simulink model "Selfmade_model_robot"  (R2024b)
settings: Solver=VariableStepAuto  StartTime=0.0  StopTime=10.0  RelTol=1e-3
values from neighbouring files (symbols this model uses):
  ua2tau = (2*gbox.N*mot.Kt/mot.R)*[1;-1]    [lab4_model_startup.m]
undefined symbols (not defined in the file or in its folder): drv, g, gbox, model, ms22g, sens, Ts, wheel
settings Model: Creator=bmm1  LastModifiedBy=pries

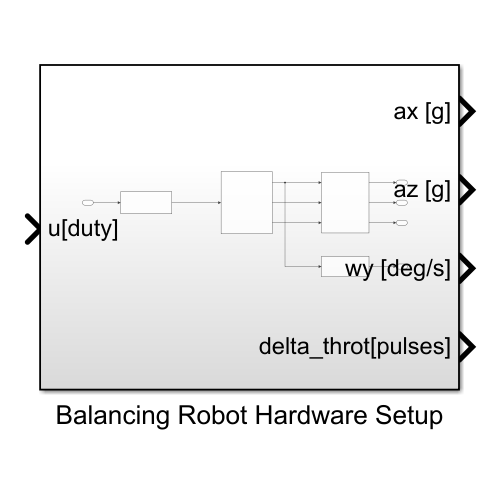
[thumbnail: Simulink's stored preview of the top-level diagram]
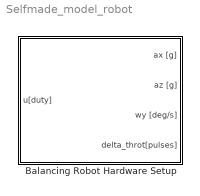
== system Selfmade_model_robot ==
  Balancing Robot Hardware Setup : Subsystem

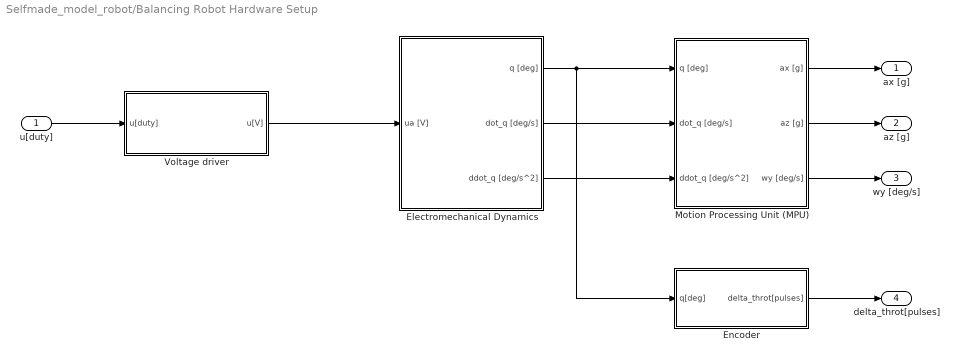
== system Selfmade_model_robot/Balancing Robot Hardware Setup ==
  u[duty] : Inport
  Electromechanical Dynamics : Subsystem
  Encoder : Subsystem
  Motion Processing Unit (MPU) : Subsystem
  Voltage driver : Subsystem
  ax [g] : Outport
  az [g] : Outport  Port=2
  wy [deg/s] : Outport  Port=3
  delta_throt[pulses] : Outport  Port=4
  wires:
  Voltage driver/1(u[V]) -> Electromechanical Dynamics/1(ua [V])
  Electromechanical Dynamics/1(q [deg]) -> Encoder/1(q[deg]), Motion Processing Unit (MPU)/1(q [deg])
  u[duty]/1 -> Voltage driver/1(u[duty])
  Electromechanical Dynamics/3(ddot_q [deg/s^2]) -> Motion Processing Unit (MPU)/3(ddot_q [deg/s^2])
  Motion Processing Unit (MPU)/3(wy [deg/s]) -> wy [deg/s]/1
  Electromechanical Dynamics/2(dot_q [deg/s]) -> Motion Processing Unit (MPU)/2(dot_q [deg/s])
  Motion Processing Unit (MPU)/2(az [g]) -> az [g]/1
  Motion Processing Unit (MPU)/1(ax [g]) -> ax [g]/1
  Encoder/1(delta_throt[pulses]) -> delta_throt[pulses]/1

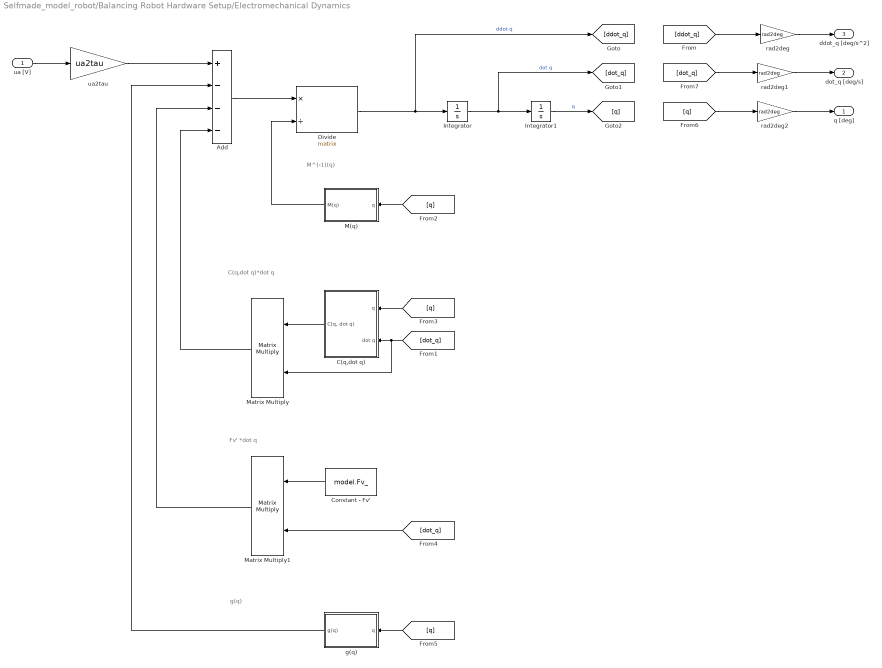
== system Selfmade_model_robot/Balancing Robot Hardware Setup/Electromechanical Dynamics ==
  note: g(q)
  note: Fv' *dot q
  note: C(q,dot q)*dot q
  note: M^(-1)(q)
  ua [V] : Inport
  Add : Sum  Inputs=+---
  C(q,dot q) : Subsystem
  Constant - Fv' : Constant  Value=model.Fv_
  Divide : Product  Inputs=*/  Multiplication=Matrix(*)
  Integrator : Integrator
  Integrator1 : Integrator
  M(q) : Subsystem
  Matrix Multiply : Product  Multiplication=Matrix(*)
  Matrix Multiply1 : Product  Multiplication=Matrix(*)
  g(q) : Subsystem
  rad2deg : Gain  Gain=rad2deg
  rad2deg1 : Gain  Gain=rad2deg
  rad2deg2 : Gain  Gain=rad2deg
  ua2tau : Gain  Gain=ua2tau
  q [deg] : Outport
  dot_q [deg/s] : Outport  Port=2
  ddot_q [deg/s^2] : Outport  Port=3
  wires:
  ua [V]/1 -> ua2tau/1
  ua2tau/1 -> Add/1
  Add/1 -> Divide/1
  Divide/1 -> [ddot_q], Integrator/1  "ddot q"
  Integrator/1 -> [dot_q], Integrator1/1  "dot q"
  Integrator1/1 -> [q]  "q"
  [q] -> M(q)/1(q)
  M(q)/1(M(q)) -> Divide/2
  C(q,dot q)/1("C(q, dot q)") -> Matrix Multiply/1
  [dot_q] -> Matrix Multiply/2, C(q,dot q)/2(dot q)
  [q] -> C(q,dot q)/1(q)
  Constant - Fv'/1 -> Matrix Multiply1/1
  [dot_q] -> Matrix Multiply1/2
  [q] -> g(q)/1(q)
  Matrix Multiply/1 -> Add/4
  Matrix Multiply1/1 -> Add/3
  g(q)/1(g(q)) -> Add/2
  [ddot_q] -> rad2deg/1
  [dot_q] -> rad2deg1/1
  [q] -> rad2deg2/1
  rad2deg2/1 -> q [deg]/1
  rad2deg/1 -> ddot_q [deg/s^2]/1
  rad2deg1/1 -> dot_q [deg/s]/1

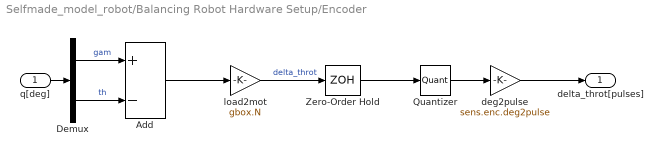
== system Selfmade_model_robot/Balancing Robot Hardware Setup/Encoder ==
  q[deg] : Inport
  Add : Sum  Inputs=+-
  Demux : Demux  Outputs=2
  Quantizer : Quantizer  QuantizationInterval=sens.enc.pulse2deg
  Zero-Order Hold : ZeroOrderHold  SampleTime=Ts
  deg2pulse : Gain  Gain=sens.enc.deg2pulse
  load2mot : Gain  Gain=gbox.N
  delta_throt[pulses] : Outport
  wires:
  Add/1 -> load2mot/1
  Zero-Order Hold/1 -> Quantizer/1
  q[deg]/1 -> Demux/1
  Demux/2 -> Add/2  "th"
  Quantizer/1 -> deg2pulse/1
  Demux/1 -> Add/1  "gam"
  deg2pulse/1 -> delta_throt[pulses]/1
  load2mot/1 -> Zero-Order Hold/1  "delta_throt"

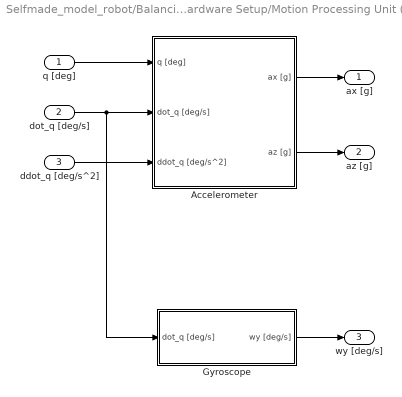
== system Selfmade_model_robot/Balancing Robot Hardware Setup/Motion Processing Unit (MPU) ==
  q [deg] : Inport
  dot_q [deg/s] : Inport  Port=2
  ddot_q [deg/s^2] : Inport  Port=3
  Accelerometer : Subsystem
  Gyroscope : Subsystem
  ax [g] : Outport
  az [g] : Outport  Port=2
  wy [deg/s] : Outport  Port=3
  wires:
  Gyroscope/1(wy [deg/s]) -> wy [deg/s]/1
  ddot_q [deg/s^2]/1 -> Accelerometer/3(ddot_q [deg/s^2])
  q [deg]/1 -> Accelerometer/1(q [deg])
  Accelerometer/1(ax [g]) -> ax [g]/1
  dot_q [deg/s]/1 -> Gyroscope/1(dot_q [deg/s]), Accelerometer/2(dot_q [deg/s])
  Accelerometer/2(az [g]) -> az [g]/1

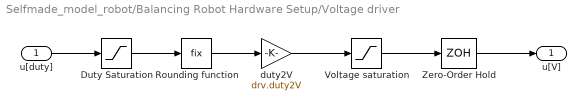
== system Selfmade_model_robot/Balancing Robot Hardware Setup/Voltage driver ==
  u[duty] : Inport
  Duty Saturation : Saturate  UpperLimit=drv.dutymax  LowerLimit=-drv.dutymax
  Rounding function : Rounding  Operator=fix
  Voltage saturation : Saturate  UpperLimit=drv.Vbus  LowerLimit=-drv.Vbus
  Zero-Order Hold : ZeroOrderHold  SampleTime=Ts
  duty2V : Gain  Gain=drv.duty2V
  u[V] : Outport
  wires:
  Voltage saturation/1 -> Zero-Order Hold/1
  duty2V/1 -> Voltage saturation/1
  Rounding function/1 -> duty2V/1
  Zero-Order Hold/1 -> u[V]/1
  Duty Saturation/1 -> Rounding function/1
  u[duty]/1 -> Duty Saturation/1

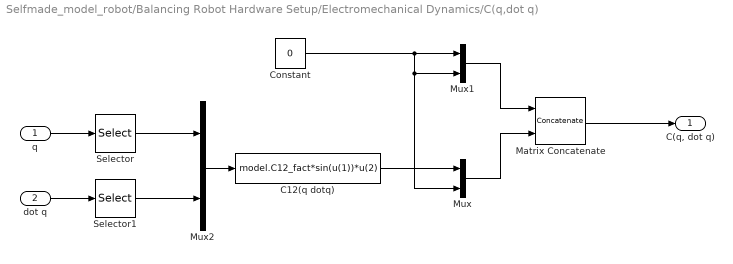
== system Selfmade_model_robot/Balancing Robot Hardware Setup/Electromechanical Dynamics/C(q,dot q) ==
  q : Inport
  dot q : Inport  Port=2
  C12(q dotq) : Fcn  Expr=model.C12_fact*sin(u(1))*u(2)
  Constant : Constant  Value=0
  Matrix Concatenate : Concatenate  Mode=Multidimensional array  ConcatenateDimension=2
  Mux : Mux  Inputs=2
  Mux1 : Mux  Inputs=2
  Mux2 : Mux  Inputs=2
  Selector : Selector  InputPortWidth=2  IndexOptions=Index vector (dialog)  Indices=2  OutputSizes=1
  Selector1 : Selector  InputPortWidth=2  IndexOptions=Index vector (dialog)  Indices=2  OutputSizes=1
  "C(q, dot q)" : Outport
  wires:
  Matrix Concatenate/1 -> "C(q, dot q)"/1
  Mux/1 -> Matrix Concatenate/2
  Mux1/1 -> Matrix Concatenate/1
  Selector/1 -> Mux2/1
  q/1 -> Selector/1
  dot q/1 -> Selector1/1
  Constant/1 -> Mux/2, Mux1/2, Mux1/1
  Selector1/1 -> Mux2/2
  Mux2/1 -> C12(q dotq)/1
  C12(q dotq)/1 -> Mux/1

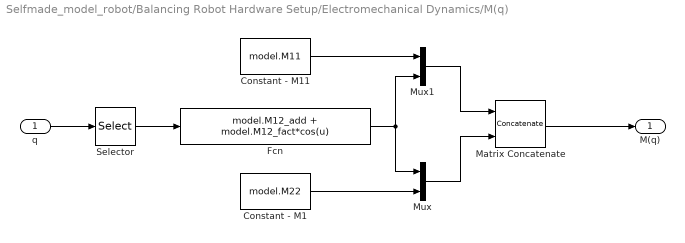
== system Selfmade_model_robot/Balancing Robot Hardware Setup/Electromechanical Dynamics/M(q) ==
  q : Inport
  Constant - M1 : Constant  Value=model.M22
  Constant - M11 : Constant  Value=model.M11
  Fcn : Fcn  Expr=model.M12_add + model.M12_fact*cos(u)
  Matrix Concatenate : Concatenate  Mode=Multidimensional array  ConcatenateDimension=2
  Mux : Mux  Inputs=2
  Mux1 : Mux  Inputs=2
  Selector : Selector  InputPortWidth=2  IndexOptions=Index vector (dialog)  Indices=2  OutputSizes=1
  M(q) : Outport
  wires:
  q/1 -> Selector/1
  Selector/1 -> Fcn/1
  Constant - M1/1 -> Mux/2
  Constant - M11/1 -> Mux1/1
  Fcn/1 -> Mux/1, Mux1/2
  Mux1/1 -> Matrix Concatenate/1
  Mux/1 -> Matrix Concatenate/2
  Matrix Concatenate/1 -> M(q)/1

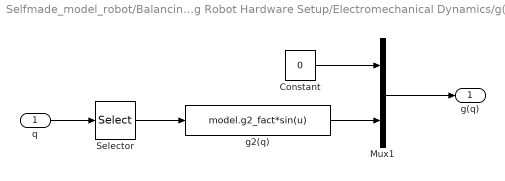
== system Selfmade_model_robot/Balancing Robot Hardware Setup/Electromechanical Dynamics/g(q) ==
  q : Inport
  Constant : Constant  Value=0
  Mux1 : Mux  Inputs=2
  Selector : Selector  InputPortWidth=2  IndexOptions=Index vector (dialog)  Indices=2  OutputSizes=1
  g2(q) : Fcn  Expr=model.g2_fact*sin(u)
  g(q) : Outport
  wires:
  Selector/1 -> g2(q)/1
  Constant/1 -> Mux1/1
  q/1 -> Selector/1
  g2(q)/1 -> Mux1/2
  Mux1/1 -> g(q)/1

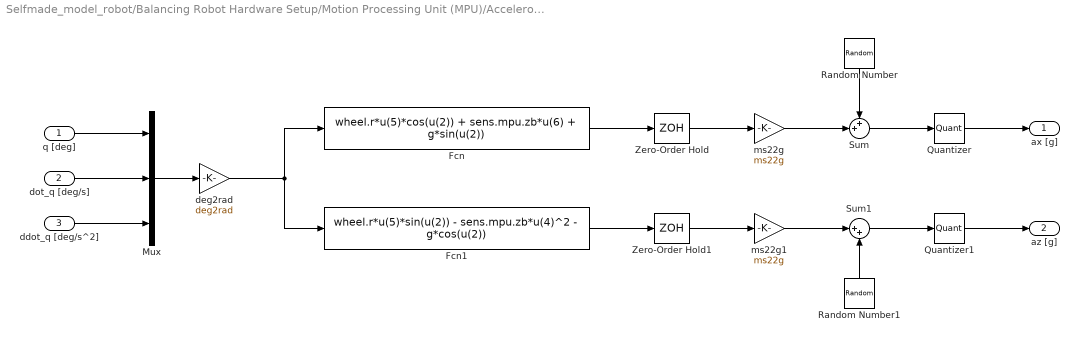
== system Selfmade_model_robot/Balancing Robot Hardware Setup/Motion Processing Unit (MPU)/Accelerometer ==
  q [deg] : Inport
  dot_q [deg/s] : Inport  Port=2
  ddot_q [deg/s^2] : Inport  Port=3
  Fcn : Fcn  Expr=wheel.r*u(5)*cos(u(2)) + sens.mpu.zb*u(6) + g*sin(u(2))
  Fcn1 : Fcn  Expr=wheel.r*u(5)*sin(u(2)) - sens.mpu.zb*u(4)^2 - g*cos(u(2))
  Mux : Mux  Inputs=3
  Quantizer : Quantizer  QuantizationInterval=sens.mpu.acc.LSB2g
  Quantizer1 : Quantizer  QuantizationInterval=sens.mpu.acc.LSB2g
  Random Number : RandomNumber  Variance=sens.mpu.acc.noisevar  SampleTime=Ts
  Random Number1 : RandomNumber  Variance=sens.mpu.acc.noisevar  SampleTime=Ts
  Sum : Sum  Inputs=++|
  Sum1 : Sum  Inputs=|++
  Zero-Order Hold : ZeroOrderHold  SampleTime=Ts
  Zero-Order Hold1 : ZeroOrderHold  SampleTime=Ts
  deg2rad : Gain  Gain=deg2rad
  ms22g : Gain  Gain=ms22g
  ms22g1 : Gain  Gain=ms22g
  ax [g] : Outport
  az [g] : Outport  Port=2
  wires:
  q [deg]/1 -> Mux/1
  dot_q [deg/s]/1 -> Mux/2
  ddot_q [deg/s^2]/1 -> Mux/3
  Mux/1 -> deg2rad/1
  deg2rad/1 -> Fcn/1, Fcn1/1
  Fcn/1 -> Zero-Order Hold/1
  Fcn1/1 -> Zero-Order Hold1/1
  Zero-Order Hold/1 -> ms22g/1
  Zero-Order Hold1/1 -> ms22g1/1
  ms22g/1 -> Sum/2
  Random Number/1 -> Sum/1
  Random Number1/1 -> Sum1/2
  ms22g1/1 -> Sum1/1
  Sum1/1 -> Quantizer1/1
  Sum/1 -> Quantizer/1
  Quantizer/1 -> ax [g]/1
  Quantizer1/1 -> az [g]/1

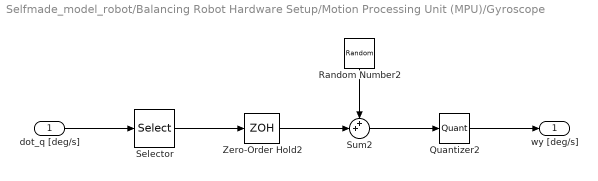
== system Selfmade_model_robot/Balancing Robot Hardware Setup/Motion Processing Unit (MPU)/Gyroscope ==
  dot_q [deg/s] : Inport
  Quantizer2 : Quantizer  QuantizationInterval=sens.mpu.gyro.LSB2g
  Random Number2 : RandomNumber  Variance=sens.mpu.gyro.noisevar  SampleTime=Ts
  Selector : Selector  InputPortWidth=2  IndexOptions=Index vector (dialog)  Indices=2  OutputSizes=1
  Sum2 : Sum  Inputs=++|
  Zero-Order Hold2 : ZeroOrderHold  SampleTime=Ts
  wy [deg/s] : Outport
  wires:
  Sum2/1 -> Quantizer2/1
  Zero-Order Hold2/1 -> Sum2/2
  Random Number2/1 -> Sum2/1
  Quantizer2/1 -> wy [deg/s]/1
  dot_q [deg/s]/1 -> Selector/1
  Selector/1 -> Zero-Order Hold2/1
